simulink model "Velocity_Controlled_Vehicle"  (R2022b)
settings: Solver=FixedStepAuto  StartTime=0.0  StopTime=T  RelTol=1e-3
values from neighbouring files (symbols this model uses):
  Ts = 0.1    [parameter.m]
settings Model: Creator=nil_c  LastModifiedBy=nils
settings OptimizationCC: EnhancedBackFolding=on  PassReuseOutputArgsThreshold=0  ZeroExternalMemoryAtStartup=off  ZeroInternalMemoryAtStartup=off  OptimizeBlockOrder=speed  DifferentSizesBufferReuse=on  OptimizationCustomize=off
settings DebuggingCC: ParameterTunabilityLossMsg=error  SFUnexpectedBacktrackingDiag=warning  SFNoUnconditionalDefaultTransitionDiag=warning
settings SFSimCC: MATLABDynamicMemAlloc=off  SimTargetLang=C++
settings RTWCC: GenerateReport=on  BuildConfiguration=Debug  LaunchReport=on  TargetLang=C++
settings CodeAppCC: ForceParamTrailComments=on  OperatorAnnotations=on  EnableCustomComments=on
settings GRTTargetCC: TargetLangStandard=C++11 (ISO)  CodeInterfacePackaging=C++ class  MultiInstanceErrorCode=None

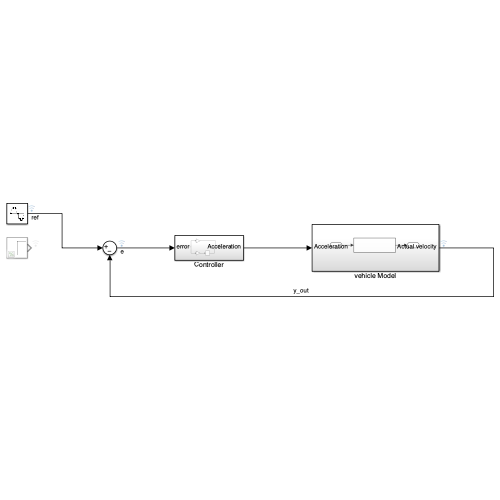
[thumbnail: Simulink's stored preview of the top-level diagram]
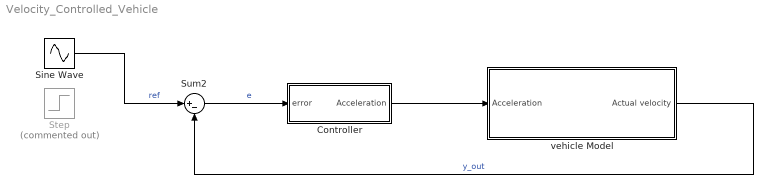
== system Velocity_Controlled_Vehicle ==
  Controller : Subsystem
      settings: RTWFcnNameOpts=Use subsystem name
  Sine Wave : Sin  Bias=30  Frequency=0.2  SampleTime=Ts
  Step : Step  Commented=on  SampleTime=Ts
  Sum2 : Sum  Inputs=|+-
  vehicle Model : Subsystem  RTWFcnName=vehicle_model
      settings: RTWFcnNameOpts=User specified
  wires:
  vehicle Model/1(Actual velocity) -> Sum2/2  "y_out"
  Sum2/1 -> Controller/1(error)  "e"
  Controller/1(Acceleration) -> vehicle Model/1(Acceleration)
  Sine Wave/1 -> Sum2/1  "ref"

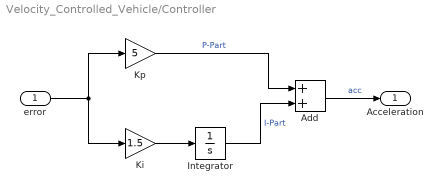
== system Velocity_Controlled_Vehicle/Controller ==
  error : Inport
  Add : Sum
  Integrator : Integrator
  Ki : Gain  Gain=1.5
  Kp : Gain  Gain=5
  Acceleration : Outport
  wires:
  Ki/1 -> Integrator/1
  Add/1 -> Acceleration/1  "acc"
  Kp/1 -> Add/1  "P-Part"
  Integrator/1 -> Add/2  "I-Part"
  error/1 -> Ki/1, Kp/1

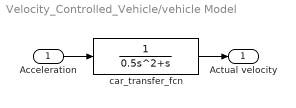
== system Velocity_Controlled_Vehicle/vehicle Model ==
  Acceleration : Inport
  car_transfer_fcn : TransferFcn  Numerator=[0 0 1]  Denominator=[0.5 1 0]
  Actual velocity : Outport  VectorParamsAs1DForOutWhenUnconnected=off
  wires:
  Acceleration/1 -> car_transfer_fcn/1
  car_transfer_fcn/1 -> Actual velocity/1
